simulink model "simpowersystems_simple_phasor"  (Simulink 7.8)
settings: Solver=FixedStepDiscrete  StartTime=0.0  StopTime=inf  FixedStep=1  MaxStep=1/60  RelTol=1e-3
InitFcn:
  | Ts = 1e-5;
undefined symbols (not defined in the file): j
libraries: powerlib x10, powerlib_extras x3, simulink x2
settings Model: Creator=sfrank1  LastModifiedBy=sfrank1
settings DebuggingCC: FcnCallInpInsideContextMsg=Use local settings

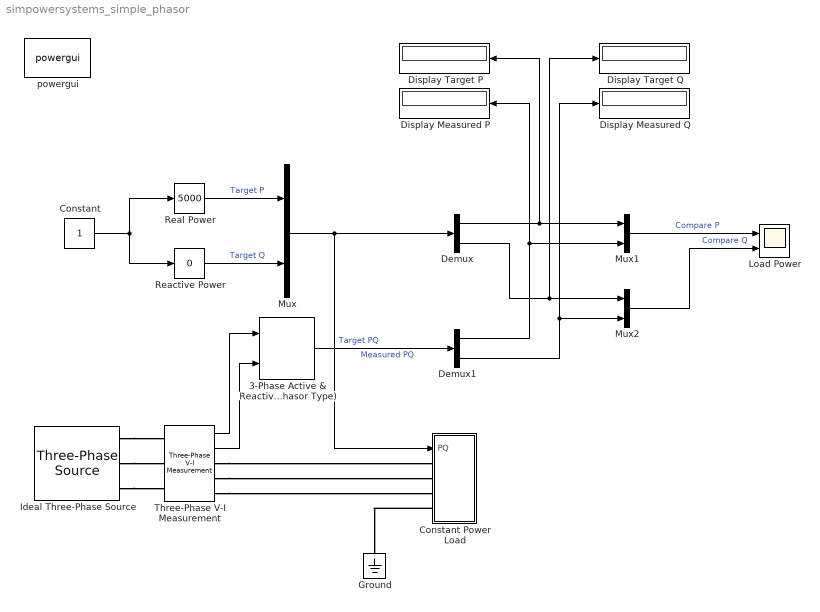
== system simpowersystems_simple_phasor ==
  3-Phase Active & Reactive Power (Phasor Type) : powerlib_extras/Phasor Library/3-Phase Active & Reactive Power (Phasor Type)
  Constant : Constant
  Constant Power Load : Subsystem  mask(Constant Power Load){PNom=5000, QNom=2000, VNom=480, fNom=60, VLow=0.7}
      mask prompts: PNom "Nominal three-phase real power (W)"; QNom "Nominal three-phase reactive power (VAR)"; VNom "Nominal line-to-line voltage (VRMS)"; fNom "Nominal frequency (Hz)"; VLow "Lower voltage limit (pu)"
      mask help: Implements a controllable constant power load, where VI* = P + jQ (in per-unit).
      mask init:
      | % Check voltages
      | if VNom <= 0
      |     error('Nominal line-to-line voltage for a constant power block must be strictly positive.');
      | end
      | if VLow <= 0
      |     error('Lower cutoff voltage for a constant power block must be strictly positive.');
      | end
      mask Help: Implements a controllable constant power load, where VI* = P + jQ (in per-unit).
  Demux : Demux  Outputs=2
  Demux1 : Demux  Outputs=2
  Display Measured P : Display
  Display Measured Q : Display
  Display Target P : Display
  Display Target Q : Display
  Ground : powerlib/Elements/Ground  LConnTagsString=a
  Ideal Three-Phase Source : powerlib/Electrical Sources/Three-Phase Source  Voltage=480  PhaseAngle=0  Frequency=60  InternalConnection=Yg  SpecifyImpedance=on  Resistance=0  Inductance=0  ShortCircuitLevel=1e6  BaseVoltage=480  XRratio=1  BusType=swing  Pref=0  Qref=0  Qmin=-inf  Qmax=inf
  Load Power : Scope  NumInputPorts=2
      settings: TickLabels=on  YMin=4880~-1  YMax=5000~1
  Mux : Mux  Inputs=2
  Mux1 : Mux  Inputs=2
  Mux2 : Mux  Inputs=2
  Reactive Power : simulink/Math Operations/Slider Gain  low=-5000  gain=0  high=5000
  Real Power : simulink/Math Operations/Slider Gain  low=0  gain=5000  high=10000
  Three-Phase V-I Measurement : powerlib/Measurements/Three-Phase V-I Measurement  VoltageMeasurement=phase-to-ground  SetLabelV=off  LabelV=Vabc  Vpu=off  VpuLL=off  CurrentMeasurement=yes  SetLabelI=off  LabelI=Iabc  Ipu=off  Pbase=100e6  Vbase=500e3  OutputType=Complex  PhasorSimulation=on  PSBequivalent=0
  powergui : powerlib/powergui  Priority=1  SimulationMode=Phasor  SolverType=Tustin  SampleTime=50e-6  frequency=60  SPID=off  DisableSnubberDevices=off  DisableRonSwitches=off  DisableVfSwitches=off  SwTol=0  Interpol=off  DisplayEquations=off  FunctionMessages=off  frequencyindice=60  Pbase=100e3  ErrMax=1e-4  Iterations=50  UnitsV=kV  UnitsW=MW  echomessages=off  HookPort=off  EnableUseOfTLC=off  x0status=blocks  RestoreLinks=warning  ResistiveCurrentMeasurement=off  Ylog=off  Xlog=on  ShowGrid=off  save=off  variable=ZData  ZoomFFT=off  StartTime=0.0  cycles=1  DisplayStyle=1  FreqAxis=off  MaxFrequency=1000  frequencyindicesteady=1  display=off  methode=off
  wires:
  Constant/1 -> Reactive Power/1, Real Power/1
  Real Power/1 -> Mux/1  "Target P"
  Mux/1 -> Constant Power Load/1(PQ), Demux/1  "Target PQ"
  Three-Phase V-I Measurement/1 -> 3-Phase Active & Reactive Power (Phasor Type)/1
  Three-Phase V-I Measurement/2 -> 3-Phase Active & Reactive Power (Phasor Type)/2
  Reactive Power/1 -> Mux/2  "Target Q"
  3-Phase Active & Reactive Power (Phasor Type)/1 -> Demux1/1  "Measured PQ"
  Mux1/1 -> Load Power/1  "Compare P"
  Mux2/1 -> Load Power/2  "Compare Q"
  Demux/1 -> Mux1/1, Display Target P/1
  Demux1/1 -> Display Measured P/1, Mux1/2
  Demux/2 -> Mux2/1, Display Target Q/1
  Demux1/2 -> Mux2/2, Display Measured Q/1
  connections:
  Ideal Three-Phase Source/RConn1 -- Three-Phase V-I Measurement/LConn1
  Ideal Three-Phase Source/RConn2 -- Three-Phase V-I Measurement/LConn2
  Ideal Three-Phase Source/RConn3 -- Three-Phase V-I Measurement/LConn3
  Three-Phase V-I Measurement/RConn3 -- Constant Power Load/LConn3
  Three-Phase V-I Measurement/RConn2 -- Constant Power Load/LConn2
  Three-Phase V-I Measurement/RConn1 -- Constant Power Load/LConn1
  Constant Power Load/LConn4 -- Ground/LConn1

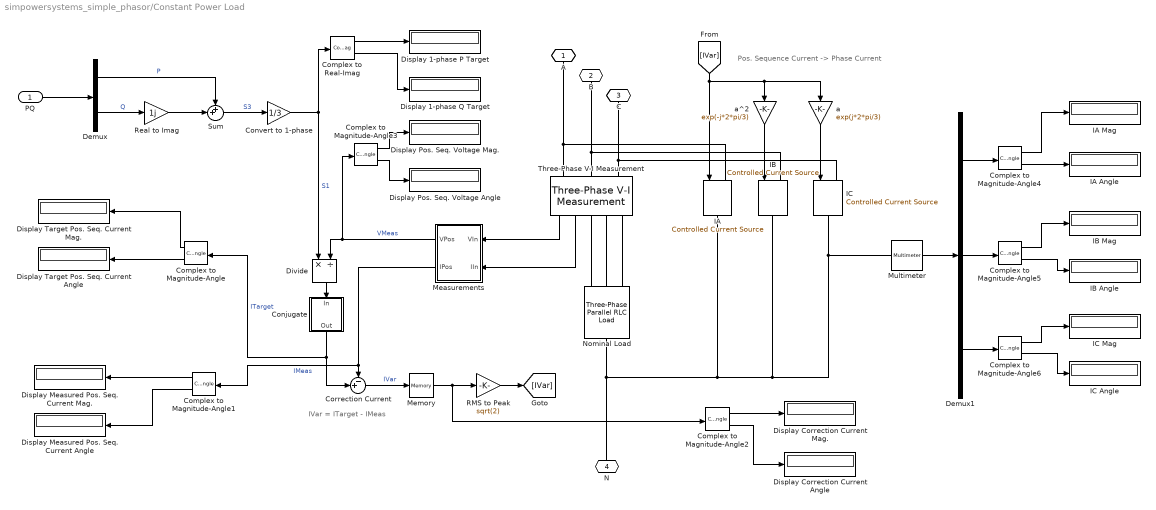
== system simpowersystems_simple_phasor/Constant Power Load ==
  note: IVar = ITarget - IMeas
  note: Pos. Sequence Current -> Phase Current
  PQ : Inport  PortDimensions=2
  Complex to Magnitude-Angle{,1..6} (7 alike) : ComplexToMagnitudeAngle
  Complex to Real-Imag : ComplexToRealImag
  Conjugate : Subsystem
  Convert to 1-phase : Gain  Gain=1/3
  Correction Current : Sum  Inputs=-+|
  Demux : Demux  Outputs=2
  Demux1 : Demux  Outputs=3
  Display 1-phase P Target : Display
  Display 1-phase Q Target : Display
  Display Correction Current Angle : Display
  Display Correction Current Mag. : Display
  Display Measured Pos. Seq. Current Angle : Display
  Display Measured Pos. Seq. Current Mag. : Display
  Display Pos. Seq. Voltage Angle : Display
  Display Pos. Seq. Voltage Mag. : Display
  Display Target Pos. Seq. Current Angle : Display
  Display Target Pos. Seq. Current Mag. : Display
  Divide : Product  Inputs=*/
  IA : powerlib/Electrical Sources/Controlled Current Source  Initialize=off  Source_Type=AC  Amplitude=0  Phase=0  Frequency=0  Measurements=Current
  IA Angle : Display
  IA Mag : Display
  IB : powerlib/Electrical Sources/Controlled Current Source  Initialize=off  Source_Type=AC  Amplitude=0  Phase=0  Frequency=0  Measurements=Current
  IB Angle : Display
  IB Mag : Display
  IC : powerlib/Electrical Sources/Controlled Current Source  Initialize=off  Source_Type=AC  Amplitude=0  Phase=0  Frequency=0  Measurements=Current
  IC Angle : Display
  IC Mag : Display
  Measurements : Subsystem
  Memory : Memory
  Multimeter : powerlib/Measurements/Multimeter  PhasorSimulation=on  OutputType=Complex  sel=[1 2 3]  L=3  Gain=[1 1 1]  yselected={'Isrc: Constant Power Load/IA','Isrc: Constant Power Load/IB','Isrc: Constant Power Load/IC'};  PSBOutputType=1  PSBequivalent=0  AxesSetting=[0,0.1,-100,100]  Display=0  SavedBlockNames=-11
  Nominal Load : powerlib/Elements/Three-Phase Parallel RLC Load  LConnTagsString=A|B|C  RConnTagsString=N  Configuration=Y (neutral)  NominalVoltage=VNom  NominalFrequency=fNom  ActivePower=PNom  InductivePower=max(QNom,0)  CapacitivePower=max(-QNom,0)  Measurements=None  LoadType=constant PQ
  RMS to Peak : Gain  Gain=sqrt(2)
  Real to Imag : Gain  Gain=1j
  Sum : Sum  Inputs=++|
  Three-Phase V-I Measurement : powerlib/Measurements/Three-Phase V-I Measurement  VoltageMeasurement=phase-to-ground  SetLabelV=off  LabelV=Vabc  Vpu=off  VpuLL=off  CurrentMeasurement=yes  SetLabelI=off  LabelI=Iabc  Ipu=off  Pbase=100e6  Vbase=VNom  OutputType=Complex  PhasorSimulation=on  PSBequivalent=0
  a : Gain  Gain=exp(j*2*pi/3)
  a^2 : Gain  Gain=exp(-j*2*pi/3)
  A : PMIOPort  Port=1  Side=Left
  B : PMIOPort  Port=2  Side=Left
  C : PMIOPort  Port=3  Side=Left
  N : PMIOPort  Port=4  Side=Left
  wires:
  Three-Phase V-I Measurement/1 -> Measurements/1(VIn)
  Three-Phase V-I Measurement/2 -> Measurements/2(IIn)
  PQ/1 -> Demux/1
  Demux/2 -> Real to Imag/1  "Q"
  Demux/1 -> Sum/1  "P"
  Real to Imag/1 -> Sum/2
  Measurements/1(VPos) -> Divide/2, Complex to Magnitude-Angle3/1  "VMeas"
  Sum/1 -> Convert to 1-phase/1  "S3"
  Convert to 1-phase/1 -> Divide/1, Complex to Real-Imag/1  "S1"
  Divide/1 -> Conjugate/1(In)
  Measurements/2(IPos) -> Correction Current/1, Complex to Magnitude-Angle1/1  "IMeas"
  [IVar] -> IA/1, a^2/1, a/1
  a^2/1 -> IB/1
  a/1 -> IC/1
  Correction Current/1 -> Memory/1  "IVar"
  Complex to Magnitude-Angle/1 -> Display Target Pos. Seq. Current Mag./1
  Complex to Magnitude-Angle/2 -> Display Target Pos. Seq. Current Angle/1
  Complex to Magnitude-Angle1/1 -> Display Measured Pos. Seq. Current Mag./1
  Complex to Magnitude-Angle1/2 -> Display Measured Pos. Seq. Current Angle/1
  Complex to Magnitude-Angle2/1 -> Display Correction Current Mag./1
  Complex to Magnitude-Angle2/2 -> Display Correction Current Angle/1
  Conjugate/1(Out) -> Correction Current/2, Complex to Magnitude-Angle/1  "ITarget"
  Complex to Real-Imag/1 -> Display 1-phase P Target/1
  Complex to Real-Imag/2 -> Display 1-phase Q Target/1
  Complex to Magnitude-Angle3/1 -> Display Pos. Seq. Voltage Mag./1
  Complex to Magnitude-Angle3/2 -> Display Pos. Seq. Voltage Angle/1
  Demux1/1 -> Complex to Magnitude-Angle4/1
  Complex to Magnitude-Angle4/1 -> IA Mag/1
  Complex to Magnitude-Angle4/2 -> IA Angle/1
  Demux1/2 -> Complex to Magnitude-Angle5/1
  Complex to Magnitude-Angle5/1 -> IB Mag/1
  Complex to Magnitude-Angle5/2 -> IB Angle/1
  Demux1/3 -> Complex to Magnitude-Angle6/1
  Complex to Magnitude-Angle6/1 -> IC Mag/1
  Complex to Magnitude-Angle6/2 -> IC Angle/1
  Multimeter/1 -> Demux1/1
  RMS to Peak/1 -> [IVar]
  Memory/1 -> Complex to Magnitude-Angle2/1, RMS to Peak/1
  connections:
  A/RConn1 -- Three-Phase V-I Measurement/LConn1 -- IA/LConn1
  B/RConn1 -- Three-Phase V-I Measurement/LConn2 -- IB/LConn1
  C/RConn1 -- Three-Phase V-I Measurement/LConn3 -- IC/LConn1
  Three-Phase V-I Measurement/RConn1 -- Nominal Load/LConn1
  Three-Phase V-I Measurement/RConn2 -- Nominal Load/LConn2
  Three-Phase V-I Measurement/RConn3 -- Nominal Load/LConn3
  IB/RConn1 -- IA/RConn1 -- Nominal Load/RConn1 -- N/RConn1 -- IC/RConn1 -- Multimeter/LConn1

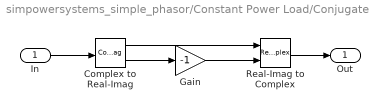
== system simpowersystems_simple_phasor/Constant Power Load/Conjugate ==
  In : Inport
  Complex to Real-Imag : ComplexToRealImag
  Gain : Gain  Gain=-1
  Real-Imag to Complex : RealImagToComplex
  Out : Outport
  wires:
  In/1 -> Complex to Real-Imag/1
  Complex to Real-Imag/1 -> Real-Imag to Complex/1
  Complex to Real-Imag/2 -> Gain/1
  Gain/1 -> Real-Imag to Complex/2
  Real-Imag to Complex/1 -> Out/1

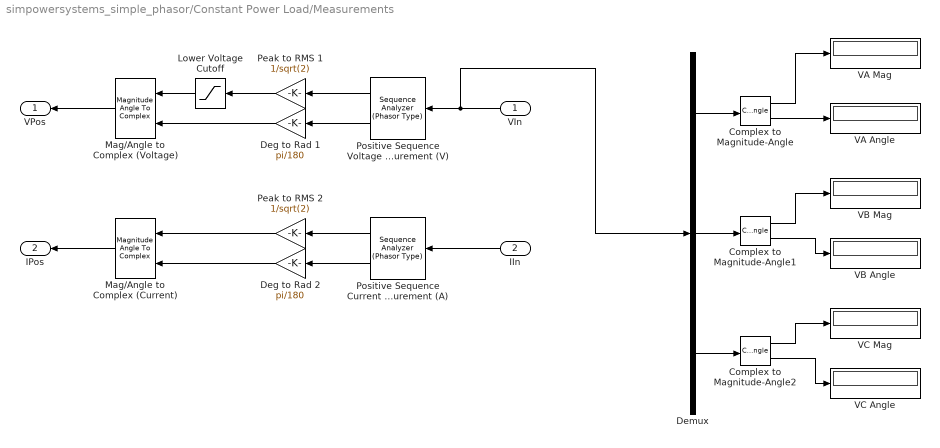
== system simpowersystems_simple_phasor/Constant Power Load/Measurements ==
  VIn : Inport
  IIn : Inport  Port=2
  Complex to Magnitude-Angle : ComplexToMagnitudeAngle
  Complex to Magnitude-Angle1 : ComplexToMagnitudeAngle
  Complex to Magnitude-Angle2 : ComplexToMagnitudeAngle
  Deg to Rad 1 : Gain  Gain=pi/180
  Deg to Rad 2 : Gain  Gain=pi/180
  Demux : Demux  Outputs=3
  Lower Voltage Cutoff : Saturate  UpperLimit=inf  LowerLimit=VLow*VNom/sqrt(3)
  Mag/Angle to Complex (Current) : MagnitudeAngleToComplex
  Mag/Angle to Complex (Voltage) : MagnitudeAngleToComplex
  Peak to RMS 1 : Gain  Gain=1/sqrt(2)
  Peak to RMS 2 : Gain  Gain=1/sqrt(2)
  Positive Sequence Current Measurement (A) : powerlib_extras/Phasor Library/Sequence Analyzer (Phasor Type)  seq=Positive
  Positive Sequence Voltage Measurement (V) : powerlib_extras/Phasor Library/Sequence Analyzer (Phasor Type)  seq=Positive
  VA Angle : Display
  VA Mag : Display
  VB Angle : Display
  VB Mag : Display
  VC Angle : Display
  VC Mag : Display
  VPos : Outport
  IPos : Outport  Port=2
  wires:
  Positive Sequence Voltage Measurement (V)/1 -> Peak to RMS 1/1
  Positive Sequence Current Measurement (A)/1 -> Peak to RMS 2/1
  Positive Sequence Current Measurement (A)/2 -> Deg to Rad 2/1
  Lower Voltage Cutoff/1 -> Mag/Angle to Complex (Voltage)/1
  VIn/1 -> Positive Sequence Voltage Measurement (V)/1, Demux/1
  IIn/1 -> Positive Sequence Current Measurement (A)/1
  Mag/Angle to Complex (Voltage)/1 -> VPos/1
  Mag/Angle to Complex (Current)/1 -> IPos/1
  Peak to RMS 1/1 -> Lower Voltage Cutoff/1
  Peak to RMS 2/1 -> Mag/Angle to Complex (Current)/1
  Demux/1 -> Complex to Magnitude-Angle/1
  Complex to Magnitude-Angle/1 -> VA Mag/1
  Complex to Magnitude-Angle/2 -> VA Angle/1
  Demux/2 -> Complex to Magnitude-Angle1/1
  Complex to Magnitude-Angle1/1 -> VB Mag/1
  Complex to Magnitude-Angle1/2 -> VB Angle/1
  Demux/3 -> Complex to Magnitude-Angle2/1
  Complex to Magnitude-Angle2/1 -> VC Mag/1
  Complex to Magnitude-Angle2/2 -> VC Angle/1
  Deg to Rad 1/1 -> Mag/Angle to Complex (Voltage)/2
  Positive Sequence Voltage Measurement (V)/2 -> Deg to Rad 1/1
  Deg to Rad 2/1 -> Mag/Angle to Complex (Current)/2
